simulink model "HQEV_MiL_20160830_integrate_2010a"  (Simulink 7.5)
settings: Solver=FixedStepDiscrete  StartTime=0.0  StopTime=inf  FixedStep=0.01  RelTol=1e-3
PostLoadFcn:
  | , if any(exist('dsrtsu_mdlpostloadfcn', 'file') == [2, 3, 6]), try dsrtsu_mdlpostloadfcn('Execute', bdroot); catch fprintf('Error in PostLoadFcn (dsrtsu_mdlpostloadfcn) for model "%s":\n %s\n', bdroot, lasterr); end, end,
values from neighbouring files (symbols this model uses):
  Bat_C_Ah = 36    [parameter_V1.mat]
  Bat_ocv_xIndex = [5 10 20 30 40 50 60 70 80 90 95]    [parameter_V1.mat]
  Bat_ocv_z = [329 332 340 345 347 351 358 372 377 386 391]    [parameter_V1.mat]
  Bat_R_ohm_z = [4.41 3.46 1.57 1.07 0.76 0.63 0.55 0.44 0.41 0.4 0.4 3.14 ... (66 elements, 11x6)]    [parameter_V1.mat]
  Bat_SOC_Init = 90    [parameter_V1.mat]
  Env_hum_pct_Ambient = 30    [parameter_V1.mat]
  Env_Slope_deg = 0    [parameter_V1.mat]
  Env_Temp_degC_Ambient = 25    [parameter_V1.mat]
  Env_v_kmph_HWind = 0    [parameter_V1.mat]
  Reducer_F_i = 7.23    [parameter_V1.mat]
  Reducer_R_i = 7.23    [parameter_V1.mat]
  Veh =     [parameter_V1.mat]
  Veh_A_m2_Fr = 2.246    [parameter_V1.mat]
  Veh_F_Brake =     [parameter_V1.mat]
  Veh_fac_AirDrag = 0.326    [parameter_V1.mat]
  Veh_fac_WhDragFrict_0 = 0.011    [parameter_V1.mat]
  Veh_g_mps2_C = 9.81    [parameter_V1.mat]
  Veh_GainBrake =     [parameter_V1.mat]
  Veh_h_m_COGHigh = 0.5    [parameter_V1.mat]
  Veh_J_kgm2_Wh = 1.3635    [parameter_V1.mat]
  Veh_L_m_AxlBas = 2.63    [parameter_V1.mat]
  Veh_M_kg = 1427    [parameter_V1.mat]
  Veh_mu_Brake = 0.4    [parameter_V1.mat]
  Veh_mu_Tyre =     [parameter_V1.mat]
  Veh_num_FrictPair = 8    [parameter_V1.mat]
  Veh_pct_Brk = 70    [parameter_V1.mat]
  Veh_r_dyn =     [parameter_V1.mat]
  Veh_r_m_BrkDisk = 0.136    [parameter_V1.mat]
  Veh_rho_kgpm3_Air = 1.2258    [parameter_V1.mat]
undefined symbols (not defined in the file or in its folder): DiscIntNeverNeededParam, p_bool_False_M, p_bool_True_M
libraries: BaseOperationLib_Browser x38, simulink x14, DTQC_lib x1, ERR_lib x1, MQM_lib x1, PTCL_lib x1, PUD_lib x1, TQD_lib x1, TQR_lib x1, VMM_lib x1, ACCA_lib x1, BBCA_lib x1
(part 14 of 15)

== system HQEV_MiL_20160830_integrate_2010a/MiL/Test_Integration/Reducer_R/FinalDrive/FinalDrive/Subsystem/Backward/Efficiency ==
  T_in : Inport
  "Temp " : Inport  Port=2
  "Omega_in " : Inport  Port=3
  Terminator : Terminator
  Terminator1 : Terminator
  Terminator2 : Terminator
  eta_constant : Constant  Value=0.94
  eta : Outport
  wires:
  "Temp "/1 -> Terminator2/1
  T_in/1 -> Terminator1/1
  "Omega_in "/1 -> Terminator/1
  eta_constant/1 -> eta/1

== system HQEV_MiL_20160830_integrate_2010a/MiL/Test_Integration/Reducer_R/FinalDrive/FinalDrive/Subsystem/Forward/Efficiency ==
  T_in : Inport
  "Temp " : Inport  Port=2
  "Omega_in " : Inport  Port=3
  Terminator : Terminator
  Terminator1 : Terminator
  Terminator2 : Terminator
  eta_constant : Constant  Value=0.94
  eta : Outport
  wires:
  "Temp "/1 -> Terminator2/1
  T_in/1 -> Terminator1/1
  "Omega_in "/1 -> Terminator/1
  eta_constant/1 -> eta/1

== system HQEV_MiL_20160830_integrate_2010a/MiL/Test_Integration/Thermal/Thermal/Subsystem/Battery_Cooling_Circle/Battery/Forced Convective ==
  note: C:specific heat capacity
  note: CQ(T2-T1)=h[T0-(T2+T1)/2]
      | T2=(hT0+CQT1-T1h/2)/(CQ+h/2)
  note: h: forced convective heat transfer coefficient
  T_Motor : Inport
  Q_water_inlet : Inport  Port=2
  T_water_inlet : Inport  Port=3
  Bus Creator : BusCreator  Inputs=5
  Bus Selector : BusSelector  OutputSignals=T_Motor,h
  Bus Selector1 : BusSelector  OutputSignals=T_Water_Inlet,Q_Water_Inlet,C
  Bus Selector2 : BusSelector  OutputSignals=T_Water_Inlet,h
  Bus Selector3 : BusSelector  OutputSignals=Q_Water_Inlet,C,h
  Bus Selector4 : BusSelector  OutputSignals=Q_Water_Inlet,C,T_Water_Inlet
  C : Constant  Value=3400
  CQT{1..8} (8 alike) : Product  RndMeth=Zero
  Const1 : Constant  Value=0.5
  Const2 : Constant  Value=0.5
  Divide1 : Product  Inputs=*/
  Scope1 : Scope
      settings: TimeRange=40  YMin=-1  YMax=1  SaveName=ScopeData22
  Scope5 : Scope
      settings: TimeRange=40  YMin=-1  YMax=1  SaveName=ScopeData21
  Subtract1 : Sum  Inputs=+-
  Subtract2 : Sum  Inputs=+-
  Unit Delay : UnitDelay  SampleTime=-1
  add2 : Sum
  add3 : Sum
  h W/deg : Constant  Value=500
  hT0 : Product  RndMeth=Zero
  q_Water2Motor : Outport
  T_water_outlet : Outport  Port=2
  Q_water_outlet : Outport  Port=3
  wires:
  T_Motor/1 -> Bus Creator/2  "T_Motor"
  T_water_inlet/1 -> Bus Creator/1  "T_Water_Inlet"
  Q_water_inlet/1 -> Bus Creator/3, Q_water_outlet/1  "Q_Water_Inlet"
  h W/deg/1 -> Bus Creator/4  "h"
  C/1 -> Bus Creator/5  "C"
  Bus Creator/1 -> Bus Selector/1, Bus Selector1/1, Bus Selector2/1, Bus Selector3/1, Bus Selector4/1
  Bus Selector/1 -> hT0/1  "<T_Motor>"
  Bus Selector/2 -> hT0/2  "<h>"
  Bus Selector1/1 -> CQT1/1  "<T_Water_Inlet>"
  Bus Selector1/2 -> CQT1/2  "<Q_Water_Inlet>"
  CQT1/1 -> CQT2/1
  Bus Selector1/3 -> CQT2/2  "<C>"
  Bus Selector2/1 -> CQT3/1  "<T_Water_Inlet>"
  Bus Selector2/2 -> CQT3/2  "<h>"
  CQT3/1 -> CQT4/1
  Const2/1 -> CQT4/2
  hT0/1 -> add2/1
  CQT2/1 -> add2/2
  add2/1 -> Subtract1/1
  CQT4/1 -> Subtract1/2
  Subtract1/1 -> Divide1/1
  Bus Selector3/1 -> CQT5/1  "<Q_Water_Inlet>"
  Bus Selector3/2 -> CQT5/2  "<C>"
  CQT5/1 -> add3/1
  Bus Selector3/3 -> CQT6/1  "<h>"
  Const1/1 -> CQT6/2
  CQT6/1 -> add3/2
  add3/1 -> Divide1/2
  Divide1/1 -> T_water_outlet/1, Unit Delay/1
  Bus Selector4/1 -> CQT7/1  "<Q_Water_Inlet>"
  Bus Selector4/2 -> CQT7/2  "<C>"
  Bus Selector4/3 -> Subtract2/1  "<T_Water_Inlet>"
  Unit Delay/1 -> Subtract2/2
  CQT7/1 -> CQT8/1, Scope5/1
  Subtract2/1 -> CQT8/2, Scope1/1
  CQT8/1 -> q_Water2Motor/1

== system HQEV_MiL_20160830_integrate_2010a/MiL/Test_Integration/Thermal/Thermal/Subsystem/Battery_Cooling_Circle/Battery/Free Convective ==
  Q_water_inlet : Inport
  T_water_inlet : Inport  Port=2
  T_water_outlet : Outport
  Q_water_outlet : Outport  Port=2
  wires:
  Q_water_inlet/1 -> Q_water_outlet/1
  T_water_inlet/1 -> T_water_outlet/1

== system HQEV_MiL_20160830_integrate_2010a/MiL/Test_Integration/Thermal/Thermal/Subsystem/Battery_Cooling_Circle/Battery/Thermal_Mass ==
  note: h: forced convective heat transfer coefficient
  note: CQ(T2-T1)=h[T0-(T2+T1)/2]
      | T2=(hT0+CQT1-T1h/2)/(CQ+h/2)
  note: C:specific heat capacity
  pwr_MotorLoss : Inport
  pwr_Water2Motor : Inport  Port=2
  BatTempIndex : Inport  Port=3
  Add : Sum
  Add1 : Sum
  C J/kg/deg : Constant  Value=450
  Compare To Constant : simulink/Logic and Bit Operations/Compare To Constant  SystemSampleTime=-1  relop===  const=0  LogicOutDataTypeMode=boolean
  Discrete-Time Integrator : DiscreteIntegrator  SampleTime=0.01  ICPrevOutput=DiscIntNeverNeededParam  ICPrevScaledInput=DiscIntNeverNeededParam
  Divide : Product  Inputs=*/
  Divide1 : Product  Inputs=*/
  Init_temp : Constant  Value=20
  Scope{,1..7} (8 alike) : Scope
      Scope settings: YMin=-1.05  YMax=-0.95  SaveName=ScopeData5
      Scope1 settings: YMin=-1.05  YMax=-0.95  SaveName=ScopeData13
      Scope2 settings: YMin=-1.05  YMax=-0.95  SaveName=ScopeData14
      Scope3 settings: YMin=-1.05  YMax=-0.95  SaveName=ScopeData15
      Scope4 settings: YMin=-1.05  YMax=-0.95  SaveName=ScopeData18
      Scope5 settings: YMin=-1.05  YMax=-0.95  SaveName=ScopeData19
      Scope6 settings: YMin=2.0625  YMax=2.11  SaveName=ScopeData20
      Scope7 settings: YMin=-1.05  YMax=-0.95  SaveName=ScopeData12
  Switch : Switch  Criteria=u2 > Threshold
  m kg : Constant  Value=200
  T_Motor : Outport
  wires:
  pwr_Water2Motor/1 -> Add/1, Scope4/1
  pwr_MotorLoss/1 -> Add/2, Scope5/1
  Add/1 -> Discrete-Time Integrator/1, Scope3/1
  Discrete-Time Integrator/1 -> Divide/1, Scope2/1
  C J/kg/deg/1 -> Divide/2
  Divide/1 -> Divide1/1, Scope1/1
  m kg/1 -> Divide1/2
  Divide1/1 -> Add1/1, Scope6/1
  Add1/1 -> T_Motor/1, Scope7/1
  BatTempIndex/1 -> Switch/3, Compare To Constant/1
  Compare To Constant/1 -> Switch/2
  Switch/1 -> Add1/2, Scope/1
  Init_temp/1 -> Switch/1

== system HQEV_MiL_20160830_integrate_2010a/MiL/Test_Integration/Thermal/Thermal/Subsystem/Battery_Cooling_Circle/Chiller/Forced Convective ==
  note: C:specific heat capacity
  note: CQ(T1-T2)=P
  note: h: forced convective heat transfer coefficient
  AC_OnOff : Inport
  Q_water_inlet : Inport  Port=2
  Temp_water_inlet : Inport  Port=3
  C J/kg/deg : Constant  Value=3400
  Divide : Product  Inputs=*/
  Product : Product  RndMeth=Zero
  Product1 : Product  RndMeth=Zero
  Saturation : Saturate  UpperLimit=inf  LowerLimit=0.5
  Subtract : Sum  Inputs=+-
  Unit Delay : UnitDelay  SampleTime=-1
  pwr_Chiller : Constant  Value=3000
  T_water_outlet : Outport
  Q_water_outlet : Outport  Port=2
  wires:
  Unit Delay/1 -> Q_water_outlet/1, Product/2
  Q_water_inlet/1 -> Unit Delay/1
  C J/kg/deg/1 -> Product/1
  Product/1 -> Saturation/1
  AC_OnOff/1 -> Product1/1
  pwr_Chiller/1 -> Product1/2
  Saturation/1 -> Divide/2
  Product1/1 -> Divide/1
  Divide/1 -> Subtract/2
  Temp_water_inlet/1 -> Subtract/1
  Subtract/1 -> T_water_outlet/1

== system HQEV_MiL_20160830_integrate_2010a/MiL/Test_Integration/Thermal/Thermal/Subsystem/Battery_Cooling_Circle/Chiller/Free Convective ==
  Q_water_inlet : Inport
  T_water_inlet : Inport  Port=2
  T_water_outlet : Outport
  Q_water_outlet : Outport  Port=2
  wires:
  Q_water_inlet/1 -> Q_water_outlet/1
  T_water_inlet/1 -> T_water_outlet/1

== system HQEV_MiL_20160830_integrate_2010a/MiL/Test_Integration/Thermal/Thermal/Subsystem/Battery_Cooling_Circle/PTC/Forced Convective ==
  note: C:specific heat capacity
  note: CQ(T1-T2)=P
  note: h: forced convective heat transfer coefficient
  PWM_PTC_pct : Inport
  Q_water_inlet : Inport  Port=2
  Temp_water_inlet : Inport  Port=3
  C : Constant
  Divide : Product  Inputs=*/
  Product : Product  RndMeth=Zero
  Product1 : Product  RndMeth=Zero
  Product2 : Product  RndMeth=Zero
  Saturation : Saturate  UpperLimit=inf  LowerLimit=0.5
  Subtract : Sum  Inputs=+-
  Unit Delay : UnitDelay  SampleTime=-1
  pct : Constant  Value=0.01
  pwr_PTC : Constant  Value=3000
  T_water_outlet : Outport
  Q_water_outlet : Outport  Port=2
  wires:
  Unit Delay/1 -> Q_water_outlet/1, Product/2
  Q_water_inlet/1 -> Unit Delay/1
  C/1 -> Product/1
  Product/1 -> Saturation/1
  pwr_PTC/1 -> Product1/2
  Saturation/1 -> Divide/2
  Product1/1 -> Divide/1
  Divide/1 -> Subtract/2
  Temp_water_inlet/1 -> Subtract/1
  Subtract/1 -> T_water_outlet/1
  PWM_PTC_pct/1 -> Product2/1
  pct/1 -> Product2/2
  Product2/1 -> Product1/1

== system HQEV_MiL_20160830_integrate_2010a/MiL/Test_Integration/Thermal/Thermal/Subsystem/Battery_Cooling_Circle/PTC/Free Convective ==
  Q_water_inlet : Inport
  T_water_inlet : Inport  Port=2
  T_water_outlet : Outport
  Q_water_outlet : Outport  Port=2
  wires:
  Q_water_inlet/1 -> Q_water_outlet/1
  T_water_inlet/1 -> T_water_outlet/1

== system HQEV_MiL_20160830_integrate_2010a/MiL/Test_Integration/Thermal/Thermal/Subsystem/Motor_Cooling_Circle/Charger/Forced Convective ==
  note: C:specific heat capacity
  note: CQ(T2-T1)=h[T0-(T2+T1)/2]
      | T2=(hT0+CQT1-T1h/2)/(CQ+h/2)
  note: h: forced convective heat transfer coefficient
  T_Motor : Inport
  Q_water_inlet : Inport  Port=2
  T_water_inlet : Inport  Port=3
  Bus Creator : BusCreator  Inputs=5
  Bus Selector : BusSelector  OutputSignals=T_Motor,h
  Bus Selector1 : BusSelector  OutputSignals=T_Water_Inlet,Q_Water_Inlet,C
  Bus Selector2 : BusSelector  OutputSignals=T_Water_Inlet,h
  Bus Selector3 : BusSelector  OutputSignals=Q_Water_Inlet,C,h
  Bus Selector4 : BusSelector  OutputSignals=Q_Water_Inlet,C,T_Water_Inlet
  C : Constant  Value=3400
  CQT{1..8} (8 alike) : Product  RndMeth=Zero
  Const1 : Constant  Value=0.5
  Const2 : Constant  Value=0.5
  Divide1 : Product  Inputs=*/
  Subtract1 : Sum  Inputs=+-
  Subtract2 : Sum  Inputs=+-
  Unit Delay : UnitDelay  SampleTime=-1
  add2 : Sum
  add3 : Sum
  h W/deg : Constant  Value=500
  hT0 : Product  RndMeth=Zero
  q_Water2Motor : Outport
  T_water_outlet : Outport  Port=2
  Q_water_outlet : Outport  Port=3
  wires:
  T_Motor/1 -> Bus Creator/2  "T_Motor"
  T_water_inlet/1 -> Bus Creator/1  "T_Water_Inlet"
  Q_water_inlet/1 -> Bus Creator/3, Q_water_outlet/1  "Q_Water_Inlet"
  h W/deg/1 -> Bus Creator/4  "h"
  C/1 -> Bus Creator/5  "C"
  Bus Creator/1 -> Bus Selector/1, Bus Selector1/1, Bus Selector2/1, Bus Selector3/1, Bus Selector4/1
  Bus Selector/1 -> hT0/1  "<T_Motor>"
  Bus Selector/2 -> hT0/2  "<h>"
  Bus Selector1/1 -> CQT1/1  "<T_Water_Inlet>"
  Bus Selector1/2 -> CQT1/2  "<Q_Water_Inlet>"
  CQT1/1 -> CQT2/1
  Bus Selector1/3 -> CQT2/2  "<C>"
  Bus Selector2/1 -> CQT3/1  "<T_Water_Inlet>"
  Bus Selector2/2 -> CQT3/2  "<h>"
  CQT3/1 -> CQT4/1
  Const2/1 -> CQT4/2
  hT0/1 -> add2/1
  CQT2/1 -> add2/2
  add2/1 -> Subtract1/1
  CQT4/1 -> Subtract1/2
  Subtract1/1 -> Divide1/1
  Bus Selector3/1 -> CQT5/1  "<Q_Water_Inlet>"
  Bus Selector3/2 -> CQT5/2  "<C>"
  CQT5/1 -> add3/1
  Bus Selector3/3 -> CQT6/1  "<h>"
  Const1/1 -> CQT6/2
  CQT6/1 -> add3/2
  add3/1 -> Divide1/2
  Divide1/1 -> T_water_outlet/1, Unit Delay/1
  Bus Selector4/1 -> CQT7/1  "<Q_Water_Inlet>"
  Bus Selector4/2 -> CQT7/2  "<C>"
  Bus Selector4/3 -> Subtract2/1  "<T_Water_Inlet>"
  Unit Delay/1 -> Subtract2/2
  CQT7/1 -> CQT8/1
  Subtract2/1 -> CQT8/2
  CQT8/1 -> q_Water2Motor/1

== system HQEV_MiL_20160830_integrate_2010a/MiL/Test_Integration/Thermal/Thermal/Subsystem/Motor_Cooling_Circle/Charger/Free Convective ==
  Q_water_inlet : Inport
  T_water_inlet : Inport  Port=2
  T_water_outlet : Outport
  Q_water_outlet : Outport  Port=2
  wires:
  Q_water_inlet/1 -> Q_water_outlet/1
  T_water_inlet/1 -> T_water_outlet/1

== system HQEV_MiL_20160830_integrate_2010a/MiL/Test_Integration/Thermal/Thermal/Subsystem/Motor_Cooling_Circle/Charger/Thermal_Mass ==
  note: h: forced convective heat transfer coefficient
  note: CQ(T2-T1)=h[T0-(T2+T1)/2]
      | T2=(hT0+CQT1-T1h/2)/(CQ+h/2)
  note: C:specific heat capacity
  pwr_MotorLoss : Inport
  pwr_Water2Motor : Inport  Port=2
  Add : Sum
  Add1 : Sum
  C J/kg/deg : Constant  Value=450
  Discrete-Time Integrator : DiscreteIntegrator  SampleTime=0.01  ICPrevOutput=DiscIntNeverNeededParam  ICPrevScaledInput=DiscIntNeverNeededParam
  Divide : Product  Inputs=*/
  Divide1 : Product  Inputs=*/
  Init_temp : Constant  Value=20
  m kg : Constant  Value=5
  T_Motor : Outport
  wires:
  pwr_Water2Motor/1 -> Add/1
  pwr_MotorLoss/1 -> Add/2
  Add/1 -> Discrete-Time Integrator/1
  Discrete-Time Integrator/1 -> Divide/1
  C J/kg/deg/1 -> Divide/2
  Divide/1 -> Divide1/1
  m kg/1 -> Divide1/2
  Divide1/1 -> Add1/1
  Init_temp/1 -> Add1/2
  Add1/1 -> T_Motor/1

== system HQEV_MiL_20160830_integrate_2010a/MiL/Test_Integration/Thermal/Thermal/Subsystem/Motor_Cooling_Circle/DCDC/Forced Convective ==
  note: C:specific heat capacity
  note: CQ(T2-T1)=h[T0-(T2+T1)/2]
      | T2=(hT0+CQT1-T1h/2)/(CQ+h/2)
  note: h: forced convective heat transfer coefficient
  T_Motor : Inport
  Q_water_inlet : Inport  Port=2
  T_water_inlet : Inport  Port=3
  Bus Creator : BusCreator  Inputs=5
  Bus Selector : BusSelector  OutputSignals=T_Motor,h
  Bus Selector1 : BusSelector  OutputSignals=T_Water_Inlet,Q_Water_Inlet,C
  Bus Selector2 : BusSelector  OutputSignals=T_Water_Inlet,h
  Bus Selector3 : BusSelector  OutputSignals=Q_Water_Inlet,C,h
  Bus Selector4 : BusSelector  OutputSignals=Q_Water_Inlet,C,T_Water_Inlet
  C : Constant  Value=3400
  CQT{1..8} (8 alike) : Product  RndMeth=Zero
  Const1 : Constant  Value=0.5
  Const2 : Constant  Value=0.5
  Divide1 : Product  Inputs=*/
  Subtract1 : Sum  Inputs=+-
  Subtract2 : Sum  Inputs=+-
  Unit Delay : UnitDelay  SampleTime=-1
  add2 : Sum
  add3 : Sum
  h W/deg : Constant  Value=500
  hT0 : Product  RndMeth=Zero
  q_Water2Motor : Outport
  T_water_outlet : Outport  Port=2
  Q_water_outlet : Outport  Port=3
  wires:
  T_Motor/1 -> Bus Creator/2  "T_Motor"
  T_water_inlet/1 -> Bus Creator/1  "T_Water_Inlet"
  Q_water_inlet/1 -> Bus Creator/3, Q_water_outlet/1  "Q_Water_Inlet"
  h W/deg/1 -> Bus Creator/4  "h"
  C/1 -> Bus Creator/5  "C"
  Bus Creator/1 -> Bus Selector/1, Bus Selector1/1, Bus Selector2/1, Bus Selector3/1, Bus Selector4/1
  Bus Selector/1 -> hT0/1  "<T_Motor>"
  Bus Selector/2 -> hT0/2  "<h>"
  Bus Selector1/1 -> CQT1/1  "<T_Water_Inlet>"
  Bus Selector1/2 -> CQT1/2  "<Q_Water_Inlet>"
  CQT1/1 -> CQT2/1
  Bus Selector1/3 -> CQT2/2  "<C>"
  Bus Selector2/1 -> CQT3/1  "<T_Water_Inlet>"
  Bus Selector2/2 -> CQT3/2  "<h>"
  CQT3/1 -> CQT4/1
  Const2/1 -> CQT4/2
  hT0/1 -> add2/1
  CQT2/1 -> add2/2
  add2/1 -> Subtract1/1
  CQT4/1 -> Subtract1/2
  Subtract1/1 -> Divide1/1
  Bus Selector3/1 -> CQT5/1  "<Q_Water_Inlet>"
  Bus Selector3/2 -> CQT5/2  "<C>"
  CQT5/1 -> add3/1
  Bus Selector3/3 -> CQT6/1  "<h>"
  Const1/1 -> CQT6/2
  CQT6/1 -> add3/2
  add3/1 -> Divide1/2
  Divide1/1 -> T_water_outlet/1, Unit Delay/1
  Bus Selector4/1 -> CQT7/1  "<Q_Water_Inlet>"
  Bus Selector4/2 -> CQT7/2  "<C>"
  Bus Selector4/3 -> Subtract2/1  "<T_Water_Inlet>"
  Unit Delay/1 -> Subtract2/2
  CQT7/1 -> CQT8/1
  Subtract2/1 -> CQT8/2
  CQT8/1 -> q_Water2Motor/1

== system HQEV_MiL_20160830_integrate_2010a/MiL/Test_Integration/Thermal/Thermal/Subsystem/Motor_Cooling_Circle/DCDC/Free Convective ==
  Q_water_inlet : Inport
  T_water_inlet : Inport  Port=2
  T_water_outlet : Outport
  Q_water_outlet : Outport  Port=2
  wires:
  Q_water_inlet/1 -> Q_water_outlet/1
  T_water_inlet/1 -> T_water_outlet/1

== system HQEV_MiL_20160830_integrate_2010a/MiL/Test_Integration/Thermal/Thermal/Subsystem/Motor_Cooling_Circle/DCDC/Thermal_Mass ==
  note: h: forced convective heat transfer coefficient
  note: CQ(T2-T1)=h[T0-(T2+T1)/2]
      | T2=(hT0+CQT1-T1h/2)/(CQ+h/2)
  note: C:specific heat capacity
  pwr_MotorLoss : Inport
  pwr_Water2Motor : Inport  Port=2
  Add : Sum
  Add1 : Sum
  C J/kg/deg : Constant  Value=450
  Discrete-Time Integrator : DiscreteIntegrator  SampleTime=0.01  ICPrevOutput=DiscIntNeverNeededParam  ICPrevScaledInput=DiscIntNeverNeededParam
  Divide : Product  Inputs=*/
  Divide1 : Product  Inputs=*/
  Init_temp : Constant  Value=20
  m kg : Constant  Value=5
  T_Motor : Outport
  wires:
  pwr_Water2Motor/1 -> Add/1
  pwr_MotorLoss/1 -> Add/2
  Add/1 -> Discrete-Time Integrator/1
  Discrete-Time Integrator/1 -> Divide/1
  C J/kg/deg/1 -> Divide/2
  Divide/1 -> Divide1/1
  m kg/1 -> Divide1/2
  Divide1/1 -> Add1/1
  Init_temp/1 -> Add1/2
  Add1/1 -> T_Motor/1

== system HQEV_MiL_20160830_integrate_2010a/MiL/Test_Integration/Thermal/Thermal/Subsystem/Motor_Cooling_Circle/Motor_F/Forced Convective ==
  note: C:specific heat capacity
  note: CQ(T2-T1)=h[T0-(T2+T1)/2]
      | T2=(hT0+CQT1-T1h/2)/(CQ+h/2)
  note: h: forced convective heat transfer coefficient
  T_Motor : Inport
  Q_water_inlet : Inport  Port=2
  T_water_inlet : Inport  Port=3
  Bus Creator : BusCreator  Inputs=5
  Bus Selector : BusSelector  OutputSignals=T_Motor,h
  Bus Selector1 : BusSelector  OutputSignals=T_Water_Inlet,Q_Water_Inlet,C
  Bus Selector2 : BusSelector  OutputSignals=T_Water_Inlet,h
  Bus Selector3 : BusSelector  OutputSignals=Q_Water_Inlet,C,h
  Bus Selector4 : BusSelector  OutputSignals=Q_Water_Inlet,C,T_Water_Inlet
  C : Constant  Value=3400
  CQT{1..8} (8 alike) : Product  RndMeth=Zero
  Const1 : Constant  Value=0.5
  Const2 : Constant  Value=0.5
  Divide1 : Product  Inputs=*/
  Subtract1 : Sum  Inputs=+-
  Subtract2 : Sum  Inputs=+-
  Unit Delay : UnitDelay  SampleTime=-1
  add2 : Sum
  add3 : Sum
  h W/deg : Constant  Value=500
  hT0 : Product  RndMeth=Zero
  q_Water2Motor : Outport
  T_water_outlet : Outport  Port=2
  Q_water_outlet : Outport  Port=3
  wires:
  T_Motor/1 -> Bus Creator/2  "T_Motor"
  T_water_inlet/1 -> Bus Creator/1  "T_Water_Inlet"
  Q_water_inlet/1 -> Bus Creator/3, Q_water_outlet/1  "Q_Water_Inlet"
  h W/deg/1 -> Bus Creator/4  "h"
  C/1 -> Bus Creator/5  "C"
  Bus Creator/1 -> Bus Selector/1, Bus Selector1/1, Bus Selector2/1, Bus Selector3/1, Bus Selector4/1
  Bus Selector/1 -> hT0/1  "<T_Motor>"
  Bus Selector/2 -> hT0/2  "<h>"
  Bus Selector1/1 -> CQT1/1  "<T_Water_Inlet>"
  Bus Selector1/2 -> CQT1/2  "<Q_Water_Inlet>"
  CQT1/1 -> CQT2/1
  Bus Selector1/3 -> CQT2/2  "<C>"
  Bus Selector2/1 -> CQT3/1  "<T_Water_Inlet>"
  Bus Selector2/2 -> CQT3/2  "<h>"
  CQT3/1 -> CQT4/1
  Const2/1 -> CQT4/2
  hT0/1 -> add2/1
  CQT2/1 -> add2/2
  add2/1 -> Subtract1/1
  CQT4/1 -> Subtract1/2
  Subtract1/1 -> Divide1/1
  Bus Selector3/1 -> CQT5/1  "<Q_Water_Inlet>"
  Bus Selector3/2 -> CQT5/2  "<C>"
  CQT5/1 -> add3/1
  Bus Selector3/3 -> CQT6/1  "<h>"
  Const1/1 -> CQT6/2
  CQT6/1 -> add3/2
  add3/1 -> Divide1/2
  Divide1/1 -> T_water_outlet/1, Unit Delay/1
  Bus Selector4/1 -> CQT7/1  "<Q_Water_Inlet>"
  Bus Selector4/2 -> CQT7/2  "<C>"
  Bus Selector4/3 -> Subtract2/1  "<T_Water_Inlet>"
  Unit Delay/1 -> Subtract2/2
  CQT7/1 -> CQT8/1
  Subtract2/1 -> CQT8/2
  CQT8/1 -> q_Water2Motor/1

== system HQEV_MiL_20160830_integrate_2010a/MiL/Test_Integration/Thermal/Thermal/Subsystem/Motor_Cooling_Circle/Motor_F/Free Convective ==
  Q_water_inlet : Inport
  T_water_inlet : Inport  Port=2
  T_water_outlet : Outport
  Q_water_outlet : Outport  Port=2
  wires:
  Q_water_inlet/1 -> Q_water_outlet/1
  T_water_inlet/1 -> T_water_outlet/1

== system HQEV_MiL_20160830_integrate_2010a/MiL/Test_Integration/Thermal/Thermal/Subsystem/Motor_Cooling_Circle/Motor_F/Thermal_Mass ==
  note: h: forced convective heat transfer coefficient
  note: CQ(T2-T1)=h[T0-(T2+T1)/2]
      | T2=(hT0+CQT1-T1h/2)/(CQ+h/2)
  note: C:specific heat capacity
  pwr_MotorLoss : Inport
  pwr_Water2Motor : Inport  Port=2
  Add : Sum
  Add1 : Sum
  C J/kg/deg : Constant  Value=450
  Discrete-Time Integrator : DiscreteIntegrator  SampleTime=0.01  ICPrevOutput=DiscIntNeverNeededParam  ICPrevScaledInput=DiscIntNeverNeededParam
  Divide : Product  Inputs=*/
  Divide1 : Product  Inputs=*/
  Init_temp : Constant  Value=20
  m kg : Constant  Value=30
  T_Motor : Outport
  wires:
  pwr_Water2Motor/1 -> Add/1
  pwr_MotorLoss/1 -> Add/2
  Add/1 -> Discrete-Time Integrator/1
  Discrete-Time Integrator/1 -> Divide/1
  C J/kg/deg/1 -> Divide/2
  Divide/1 -> Divide1/1
  m kg/1 -> Divide1/2
  Divide1/1 -> Add1/1
  Init_temp/1 -> Add1/2
  Add1/1 -> T_Motor/1

== system HQEV_MiL_20160830_integrate_2010a/MiL/Test_Integration/Thermal/Thermal/Subsystem/Motor_Cooling_Circle/Motor_R/Forced Convective ==
  note: C:specific heat capacity
  note: CQ(T2-T1)=h[T0-(T2+T1)/2]
      | T2=(hT0+CQT1-T1h/2)/(CQ+h/2)
  note: h: forced convective heat transfer coefficient
  T_Motor : Inport
  Q_water_inlet : Inport  Port=2
  T_water_inlet : Inport  Port=3
  Bus Creator : BusCreator  Inputs=5
  Bus Selector : BusSelector  OutputSignals=T_Motor,h
  Bus Selector1 : BusSelector  OutputSignals=T_Water_Inlet,Q_Water_Inlet,C
  Bus Selector2 : BusSelector  OutputSignals=T_Water_Inlet,h
  Bus Selector3 : BusSelector  OutputSignals=Q_Water_Inlet,C,h
  Bus Selector4 : BusSelector  OutputSignals=Q_Water_Inlet,C,T_Water_Inlet
  C : Constant  Value=3400
  CQT{1..8} (8 alike) : Product  RndMeth=Zero
  Const1 : Constant  Value=0.5
  Const2 : Constant  Value=0.5
  Divide1 : Product  Inputs=*/
  Subtract1 : Sum  Inputs=+-
  Subtract2 : Sum  Inputs=+-
  Unit Delay : UnitDelay  SampleTime=-1
  add2 : Sum
  add3 : Sum
  h W/deg : Constant  Value=500
  hT0 : Product  RndMeth=Zero
  q_Water2Motor : Outport
  T_water_outlet : Outport  Port=2
  Q_water_outlet : Outport  Port=3
  wires:
  T_Motor/1 -> Bus Creator/2  "T_Motor"
  T_water_inlet/1 -> Bus Creator/1  "T_Water_Inlet"
  Q_water_inlet/1 -> Bus Creator/3, Q_water_outlet/1  "Q_Water_Inlet"
  h W/deg/1 -> Bus Creator/4  "h"
  C/1 -> Bus Creator/5  "C"
  Bus Creator/1 -> Bus Selector/1, Bus Selector1/1, Bus Selector2/1, Bus Selector3/1, Bus Selector4/1
  Bus Selector/1 -> hT0/1  "<T_Motor>"
  Bus Selector/2 -> hT0/2  "<h>"
  Bus Selector1/1 -> CQT1/1  "<T_Water_Inlet>"
  Bus Selector1/2 -> CQT1/2  "<Q_Water_Inlet>"
  CQT1/1 -> CQT2/1
  Bus Selector1/3 -> CQT2/2  "<C>"
  Bus Selector2/1 -> CQT3/1  "<T_Water_Inlet>"
  Bus Selector2/2 -> CQT3/2  "<h>"
  CQT3/1 -> CQT4/1
  Const2/1 -> CQT4/2
  hT0/1 -> add2/1
  CQT2/1 -> add2/2
  add2/1 -> Subtract1/1
  CQT4/1 -> Subtract1/2
  Subtract1/1 -> Divide1/1
  Bus Selector3/1 -> CQT5/1  "<Q_Water_Inlet>"
  Bus Selector3/2 -> CQT5/2  "<C>"
  CQT5/1 -> add3/1
  Bus Selector3/3 -> CQT6/1  "<h>"
  Const1/1 -> CQT6/2
  CQT6/1 -> add3/2
  add3/1 -> Divide1/2
  Divide1/1 -> T_water_outlet/1, Unit Delay/1
  Bus Selector4/1 -> CQT7/1  "<Q_Water_Inlet>"
  Bus Selector4/2 -> CQT7/2  "<C>"
  Bus Selector4/3 -> Subtract2/1  "<T_Water_Inlet>"
  Unit Delay/1 -> Subtract2/2
  CQT7/1 -> CQT8/1
  Subtract2/1 -> CQT8/2
  CQT8/1 -> q_Water2Motor/1

== system HQEV_MiL_20160830_integrate_2010a/MiL/Test_Integration/Thermal/Thermal/Subsystem/Motor_Cooling_Circle/Motor_R/Free Convective ==
  Q_water_inlet : Inport
  T_water_inlet : Inport  Port=2
  T_water_outlet : Outport
  Q_water_outlet : Outport  Port=2
  wires:
  Q_water_inlet/1 -> Q_water_outlet/1
  T_water_inlet/1 -> T_water_outlet/1

== system HQEV_MiL_20160830_integrate_2010a/MiL/Test_Integration/Thermal/Thermal/Subsystem/Motor_Cooling_Circle/Motor_R/Thermal_Mass ==
  note: h: forced convective heat transfer coefficient
  note: CQ(T2-T1)=h[T0-(T2+T1)/2]
      | T2=(hT0+CQT1-T1h/2)/(CQ+h/2)
  note: C:specific heat capacity
  pwr_MotorLoss : Inport
  pwr_Water2Motor : Inport  Port=2
  Add : Sum
  Add1 : Sum
  C J/kg/deg : Constant  Value=450
  Discrete-Time Integrator : DiscreteIntegrator  SampleTime=0.01  ICPrevOutput=DiscIntNeverNeededParam  ICPrevScaledInput=DiscIntNeverNeededParam
  Divide : Product  Inputs=*/
  Divide1 : Product  Inputs=*/
  Init_temp : Constant  Value=20
  m kg : Constant  Value=30
  T_Motor : Outport
  wires:
  pwr_Water2Motor/1 -> Add/1
  pwr_MotorLoss/1 -> Add/2
  Add/1 -> Discrete-Time Integrator/1
  Discrete-Time Integrator/1 -> Divide/1
  C J/kg/deg/1 -> Divide/2
  Divide/1 -> Divide1/1
  m kg/1 -> Divide1/2
  Divide1/1 -> Add1/1
  Init_temp/1 -> Add1/2
  Add1/1 -> T_Motor/1

== system HQEV_MiL_20160830_integrate_2010a/MiL/Test_Integration/Thermal/Thermal/Subsystem/Motor_Cooling_Circle/Radiator/Forced Convective ==
  note: h: forced convective heat transfer coefficient
  note: CQ(T2-T1)=h[T0-(T2+T1)/2]
      | T2=(hT0+CQT1-T1h/2)/(CQ+h/2)
  note: C:specific heat capacity
  PWM_Fan : Inport
  Q_water_inlet : Inport  Port=2
  T_water_inlet : Inport  Port=3
  Bus Creator : BusCreator  Inputs=5
  Bus Selector : BusSelector  OutputSignals=T_Motor,h
  Bus Selector1 : BusSelector  OutputSignals=T_Water_Inlet,Q_Water_Inlet,C
  Bus Selector2 : BusSelector  OutputSignals=T_Water_Inlet,h
  Bus Selector3 : BusSelector  OutputSignals=Q_Water_Inlet,C,h
  C J/kg/deg : Constant  Value=3400
  CQT{1..8} (8 alike) : Product  RndMeth=Zero
  Const1 : Constant  Value=0.5
  Const2 : Constant  Value=0.5
  Const3 : Constant  Value=0.01
  Divide1 : Product  Inputs=*/
  Env_Temp_Air : Constant  Value=25
  Saturation : Saturate  UpperLimit=inf  LowerLimit=0.1
  Subtract1 : Sum  Inputs=+-
  add2 : Sum
  add3 : Sum
  h W/deg : Constant  Value=3000
  hT0 : Product  RndMeth=Zero
  T_water_outlet : Outport
  Q_water_outlet : Outport  Port=2
  wires:
  Divide1/1 -> T_water_outlet/1
  add3/1 -> Saturation/1
  CQT6/1 -> add3/2
  Const1/1 -> CQT6/2
  Bus Selector3/3 -> CQT6/1  "<h>"
  CQT5/1 -> add3/1
  Bus Selector3/2 -> CQT5/2  "<C>"
  Bus Selector3/1 -> CQT5/1  "<Q_Water_Inlet>"
  Subtract1/1 -> Divide1/1
  CQT4/1 -> Subtract1/2
  add2/1 -> Subtract1/1
  CQT2/1 -> add2/2
  hT0/1 -> add2/1
  Const2/1 -> CQT4/2
  CQT3/1 -> CQT4/1
  Bus Selector2/2 -> CQT3/2  "<h>"
  Bus Selector2/1 -> CQT3/1  "<T_Water_Inlet>"
  Bus Selector1/3 -> CQT2/2  "<C>"
  CQT1/1 -> CQT2/1
  Bus Selector1/2 -> CQT1/2  "<Q_Water_Inlet>"
  Bus Selector1/1 -> CQT1/1  "<T_Water_Inlet>"
  Bus Selector/2 -> hT0/2  "<h>"
  Bus Selector/1 -> hT0/1  "<T_Motor>"
  Bus Creator/1 -> Bus Selector2/1, Bus Selector3/1, Bus Selector1/1, Bus Selector/1
  C J/kg/deg/1 -> Bus Creator/5  "C"
  Q_water_inlet/1 -> Bus Creator/3, Q_water_outlet/1  "Q_Water_Inlet"
  T_water_inlet/1 -> Bus Creator/1  "T_Water_Inlet"
  Env_Temp_Air/1 -> Bus Creator/2  "T_Motor"
  PWM_Fan/1 -> CQT7/1
  Const3/1 -> CQT7/2
  CQT7/1 -> CQT8/1
  h W/deg/1 -> CQT8/2
  CQT8/1 -> Bus Creator/4  "h"
  Saturation/1 -> Divide1/2

== system HQEV_MiL_20160830_integrate_2010a/MiL/Test_Integration/Thermal/Thermal/Subsystem/Motor_Cooling_Circle/Radiator/Free Convective ==
  Q_water_inlet : Inport
  T_water_inlet : Inport  Port=2
  T_water_outlet : Outport
  Q_water_outlet : Outport  Port=2
  wires:
  Q_water_inlet/1 -> Q_water_outlet/1
  T_water_inlet/1 -> T_water_outlet/1

== system HQEV_MiL_20160830_integrate_2010a/MiL/Test_Integration/Vehicle/Vehicle/Vehicle/Wheel Torque/maximal_wheel_torque/F_to_T ==
  F_normal [N] : Inport
  mu_Tyre : Gain  Gain=Veh_mu_Tyre.z  SaturateOnIntegerOverflow=on  OutDataTypeStr=Inherit: Same as input  ParamDataTypeStr=Inherit: Same as input
  r_dyn : Gain  Gain=Veh_r_dyn.z  SaturateOnIntegerOverflow=on  OutDataTypeStr=Inherit: Same as input  ParamDataTypeStr=Inherit: Same as input
  T_max [Nm] : Outport
  wires:
  mu_Tyre/1 -> r_dyn/1
  F_normal [N]/1 -> mu_Tyre/1
  r_dyn/1 -> T_max [Nm]/1

== system HQEV_MiL_20160830_integrate_2010a/MiL/Test_Integration/Vehicle/Vehicle/Vehicle/Wheel Torque/maximal_wheel_torque/F_to_T_ ==
  F_normal [N] : Inport
  mu_Tyre : Gain  Gain=Veh_mu_Tyre.z  SaturateOnIntegerOverflow=on  OutDataTypeStr=Inherit: Same as input  ParamDataTypeStr=Inherit: Same as input
  r_dyn : Gain  Gain=Veh_r_dyn.z  SaturateOnIntegerOverflow=on  OutDataTypeStr=Inherit: Same as input  ParamDataTypeStr=Inherit: Same as input
  T_max [Nm] : Outport
  wires:
  r_dyn/1 -> T_max [Nm]/1
  F_normal [N]/1 -> mu_Tyre/1
  mu_Tyre/1 -> r_dyn/1

== system HQEV_MiL_20160830_integrate_2010a/MiL/Test_Integration/Vehicle/Vehicle/Vehicle/Wheel Torque/maximal_wheel_torque/Normal_force ==
  note: COG to front axle
  note: COG to rear axle
  note: COG to ground
  note: gravity aceleration
  note: wheel base
  acc_Vehicle [m/s^2] : Inport
  phi_Slope [deg] : Inport  Port=2
  m [kg] : Inport  Port=3
  Add : Sum  Inputs=+-
  Add1 : Sum
  Add2 : Sum
  Constant1 : Constant  Value=Veh_g_mps2_C
  Constant4 : Constant  Value=Veh_L_m_AxlBas
  Constant5 : Constant  Value=Veh.L_m_COGFr
  Constant6 : Constant  Value=Veh.L_m_COGRear
  Constant7 : Constant  Value=Veh_h_m_COGHigh
  Divide1 : Product  Inputs=/***
  Divide2 : Product  Inputs=/**
  Divide3 : Product  Inputs=/***
  Product : Product  RndMeth=Zero
  Product1 : Product  RndMeth=Zero
  Product2 : Product  RndMeth=Zero
  Trigonometric Function : Trigonometry  Operator=cos
  Trigonometric Function1 : Trigonometry
  deg_rad : Gain  Gain=pi/180  SaturateOnIntegerOverflow=on  OutDataTypeStr=Inherit: Same as input  ParamDataTypeStr=Inherit: Same as input
  F_normalFront [N] : Outport
  F_normalRear [N] : Outport  Port=2
  wires:
  Product2/1 -> Add2/1
  Trigonometric Function1/1 -> Product2/2
  Add2/1 -> Divide2/3
  Constant4/1 -> Divide1/1, Divide2/1, Divide3/1
  Constant6/1 -> Divide3/2
  Constant5/1 -> Divide1/2
  Constant7/1 -> Divide2/2
  acc_Vehicle [m/s^2]/1 -> Add2/2
  Constant1/1 -> Product2/1, Divide1/3, Divide3/3
  Divide1/1 -> Add1/1
  Divide2/1 -> Add/2, Add1/2
  Divide3/1 -> Add/1
  Add1/1 -> Product/2
  Add/1 -> Product1/2
  Product/1 -> F_normalRear [N]/1
  Product1/1 -> F_normalFront [N]/1
  Trigonometric Function/1 -> Divide1/4, Divide3/4
  deg_rad/1 -> Trigonometric Function1/1, Trigonometric Function/1
  phi_Slope [deg]/1 -> deg_rad/1
  m [kg]/1 -> Product/1, Product1/1

== system HQEV_MiL_20160830_integrate_2010a/MiL/Test_Integration/Charger/Charger/Charger/Charger/Work/Subsystem/AC_Charge ==
  HCU_ChargePermission : Inport
  BMS_MainPosContactorState : Inport  Port=2
  HCU_ChargeHeatingPermission : Inport  Port=3
  BMS_MainNegContactorState : Inport  Port=4
  BMS_PreChargeContactorState : Inport  Port=5
  BMS_ChargePosContactorState : Inport  Port=6
  BMS_ChargeNegContactorState : Inport  Port=7
  Bus Creator : BusCreator  Inputs=2
  Bus Creator1 : BusCreator  Inputs=2
  Bus Creator2 : BusCreator  Inputs=2
  Bus Selector : BusSelector  OutputSignals=signal1,signal2
  Charger_I : Constant  Value=0
  Charger_I1 : Constant  Value=10
  Charger_I2 : Constant  Value=5
  Charger_U : Constant  Value=0
  Charger_U1 : Constant  Value=360
  Charger_U2 : Constant  Value=360
  Logical Operator : Logic  Operator=OR  AllPortsSameDT=off  OutDataTypeMode=boolean  OutDataTypeStr=boolean
  Logical Operator1 : Logic  AllPortsSameDT=off  OutDataTypeMode=boolean  OutDataTypeStr=boolean
  Logical Operator3 : Logic  AllPortsSameDT=off  OutDataTypeMode=boolean  OutDataTypeStr=boolean
  Switch : Switch  Criteria=u2 ~= 0
  Switch1 : Switch  Criteria=u2 ~= 0
  Terminator : Terminator
  Terminator1 : Terminator
  Terminator2 : Terminator
  ChargerOutputVoltage : Outport
  ChargerOutputCurrent : Outport  Port=2
  wires:
  BMS_PreChargeContactorState/1 -> Terminator/1
  BMS_ChargePosContactorState/1 -> Terminator1/1
  BMS_ChargeNegContactorState/1 -> Terminator2/1
  HCU_ChargePermission/1 -> Logical Operator/1, Logical Operator3/2
  HCU_ChargeHeatingPermission/1 -> Logical Operator/2
  Logical Operator/1 -> Switch/2
  Charger_U/1 -> Bus Creator/1
  Charger_I/1 -> Bus Creator/2
  Bus Creator/1 -> Switch/3
  BMS_MainPosContactorState/1 -> Logical Operator1/1
  BMS_MainNegContactorState/1 -> Logical Operator1/2
  Logical Operator1/1 -> Logical Operator3/1
  Logical Operator3/1 -> Switch1/2
  Charger_U1/1 -> Bus Creator1/1
  Charger_I1/1 -> Bus Creator1/2
  Bus Creator1/1 -> Switch1/1
  Charger_U2/1 -> Bus Creator2/1
  Charger_I2/1 -> Bus Creator2/2
  Bus Creator2/1 -> Switch1/3
  Switch1/1 -> Switch/1
  Switch/1 -> Bus Selector/1
  Bus Selector/1 -> ChargerOutputVoltage/1  "<signal1>"
  Bus Selector/2 -> ChargerOutputCurrent/1  "<signal2>"

== system HQEV_MiL_20160830_integrate_2010a/MiL/Test_Integration/Charger/Charger/Charger/Charger/Work/Subsystem/Constant ==
  Constant1 : Constant  Value=30
  Constant2 : Constant
  Constant5 : Constant  Value=0
  ChargerStatus : Outport
  RechargeRequest : Outport  Port=2
  ChargerTemperature : Outport  Port=3
  wires:
  Constant2/1 -> ChargerStatus/1
  Constant5/1 -> RechargeRequest/1
  Constant1/1 -> ChargerTemperature/1

== system HQEV_MiL_20160830_integrate_2010a/MiL/Test_Integration/Driver/Driver/Driver_AutoPedal/CTRL BrakePed/velocoty/Run_Forward/Difference ==
  In1 : Inport
  Sum2 : Sum  Inputs=+-|
  Unit Delay : UnitDelay  SampleTime=-1
  Out1 : Outport
  wires:
  Sum2/1 -> Out1/1  "Gradient"
  In1/1 -> Unit Delay/1, Sum2/1
  Unit Delay/1 -> Sum2/2

== system HQEV_MiL_20160830_integrate_2010a/MiL/Test_Integration/MCU_FF/MCU/MCU/Torque_Control/Subsystem/Max_Torque/Max_Gen_Torque_Subsystem ==
  EM_Volt : Inport
  EM_spd : Inport  Port=2
  Bus Creator : BusCreator  Inputs=3
  Constant : Constant  Value=-1
  Constant1 : Constant  Value=-1
  Constant2 : Constant  Value=-1
  Interpolation_2nd : Subsystem
  Max_Gen_Torque_at_300V : Lookup  InputValues=|  Table=|  LookUpMeth=Interpolation-Use End Values
      InputValues=|
      | [0
      | 500
      | 1000
      | 1500
      | 2000
      | 2500
      | 2700
      | 3000
      | 3500
      | 4000
      | 4500
      | 5000
      | 5500
      | 6000
      | 6500
      | 7000
      | 7500
      | 8000
      | 8500
      | 9000
      | 9500
      | 10000
      | 10500
      | 11000
      | 11500
      | 12000
      | ]
      Table=|
      | [340
      | 340
      | 340
      | 340
      | 340
      | 340
      | 340
      | 316
      | 272
      | 236
      | 206
      | 180
      | 160
      | 144
      | 130
      | 120
      | 110
      | 102
      | 94
      | 88
      | 84
      | 78
      | 74
      | 70
      | 66
      | 64
      | ]
  Max_Gen_Torque_at_340V : Lookup  InputValues=|  Table=|  LookUpMeth=Interpolation-Use End Values
      InputValues=|
      | [0
      | 500
      | 1000
      | 1500
      | 2000
      | 2500
      | 3000
      | 3100
      | 3500
      | 4000
      | 4500
      | 5000
      | 5500
      | 6000
      | 6500
      | 7000
      | 7500
      | 8000
      | 8500
      | 9000
      | 9500
      | 10000
      | 10500
      | 11000
      | 11500
      | 12000
      | ]
      Table=|
      | [340
      | 340
      | 340
      | 340
      | 340
      | 340
      | 340
      | 340
      | 310
      | 272
      | 240
      | 212
      | 190
      | 170
      | 154
      | 140
      | 128
      | 118
      | 110
      | 104
      | 96
      | 90
      | 86
      | 82
      | 78
      | 74
      | ]
  Max_Mot_Torque_at_280V : Lookup  InputValues=|  Table=|  LookUpMeth=Interpolation-Use End Values
      InputValues=|
      | [0
      | 500
      | 1000
      | 1500
      | 2000
      | 2500
      | 3000
      | 3500
      | 4000
      | 4500
      | 5000
      | 5500
      | 6000
      | 6500
      | 7000
      | 7500
      | 8000
      | 8500
      | 9000
      | 9500
      | 10000
      | 10500
      | 11000
      | 11500
      | 12000
      | ]
      Table=|
      | [340
      | 340
      | 340
      | 340
      | 340
      | 340
      | 296
      | 252
      | 218
      | 188
      | 166
      | 146
      | 132
      | 120
      | 110
      | 102
      | 94
      | 88
      | 82
      | 76
      | 72
      | 68
      | 64
      | 62
      | 58
      | ]
  Product : Product  RndMeth=Zero
  Product1 : Product  RndMeth=Zero
  Product2 : Product  RndMeth=Zero
  abs_val : Subsystem
  Out1 : Outport
  wires:
  Interpolation_2nd/1(Out1) -> Out1/1
  EM_spd/1 -> abs_val/1(In1)
  Bus Creator/1 -> Interpolation_2nd/2(In2)
  EM_Volt/1 -> Interpolation_2nd/1(In1)
  abs_val/1(Out1) -> Max_Gen_Torque_at_340V/1, Max_Gen_Torque_at_300V/1, Max_Mot_Torque_at_280V/1
  Max_Mot_Torque_at_280V/1 -> Product/1
  Max_Gen_Torque_at_300V/1 -> Product1/1
  Max_Gen_Torque_at_340V/1 -> Product2/1
  Constant/1 -> Product/2
  Constant1/1 -> Product1/2
  Constant2/1 -> Product2/2
  Product/1 -> Bus Creator/1  "at280V"
  Product1/1 -> Bus Creator/2  "at300V"
  Product2/1 -> Bus Creator/3  "at340V"

== system HQEV_MiL_20160830_integrate_2010a/MiL/Test_Integration/MCU_FF/MCU/MCU/Torque_Control/Subsystem/Max_Torque/Max_Mot_Torque_Subsystem ==
  EM_Volt : Inport
  EM_spd : Inport  Port=2
  Bus Creator : BusCreator  Inputs=3
  Interpolation_2nd : Subsystem
  Max_Gen_Torque_at_300V : Lookup  InputValues=|  Table=|  LookUpMeth=Interpolation-Use End Values
      InputValues=|
      | [0
      | 500
      | 1000
      | 1500
      | 2000
      | 2500
      | 2700
      | 3000
      | 3500
      | 4000
      | 4500
      | 5000
      | 5500
      | 6000
      | 6500
      | 7000
      | 7500
      | 8000
      | 8500
      | 9000
      | 9500
      | 10000
      | 10500
      | 11000
      | 11500
      | 12000
      | ]
      Table=|
      | [340
      | 340
      | 340
      | 340
      | 340
      | 340
      | 340
      | 316
      | 272
      | 236
      | 206
      | 180
      | 160
      | 144
      | 130
      | 120
      | 110
      | 102
      | 94
      | 88
      | 84
      | 78
      | 74
      | 70
      | 66
      | 64
      | ]
  Max_Gen_Torque_at_340V : Lookup  InputValues=|  Table=|  LookUpMeth=Interpolation-Use End Values
      InputValues=|
      | [0
      | 500
      | 1000
      | 1500
      | 2000
      | 2500
      | 3000
      | 3100
      | 3500
      | 4000
      | 4500
      | 5000
      | 5500
      | 6000
      | 6500
      | 7000
      | 7500
      | 8000
      | 8500
      | 9000
      | 9500
      | 10000
      | 10500
      | 11000
      | 11500
      | 12000
      | ]
      Table=|
      | [340
      | 340
      | 340
      | 340
      | 340
      | 340
      | 340
      | 340
      | 310
      | 272
      | 240
      | 212
      | 190
      | 170
      | 154
      | 140
      | 128
      | 118
      | 110
      | 104
      | 96
      | 90
      | 86
      | 82
      | 78
      | 74
      | ]
  Max_Mot_Torque_at_280V : Lookup  InputValues=|  Table=|  LookUpMeth=Interpolation-Use End Values
      InputValues=|
      | [0
      | 500
      | 1000
      | 1500
      | 2000
      | 2500
      | 3000
      | 3500
      | 4000
      | 4500
      | 5000
      | 5500
      | 6000
      | 6500
      | 7000
      | 7500
      | 8000
      | 8500
      | 9000
      | 9500
      | 10000
      | 10500
      | 11000
      | 11500
      | 12000
      | ]
      Table=|
      | [340
      | 340
      | 340
      | 340
      | 340
      | 340
      | 296
      | 252
      | 218
      | 188
      | 166
      | 146
      | 132
      | 120
      | 110
      | 102
      | 94
      | 88
      | 82
      | 76
      | 72
      | 68
      | 64
      | 62
      | 58
      | ]
  abs_val : Subsystem
  Out1 : Outport
  wires:
  abs_val/1(Out1) -> Max_Mot_Torque_at_280V/1, Max_Gen_Torque_at_300V/1, Max_Gen_Torque_at_340V/1
  Max_Mot_Torque_at_280V/1 -> Bus Creator/1  "at280V"
  Max_Gen_Torque_at_300V/1 -> Bus Creator/2  "at300V"
  Max_Gen_Torque_at_340V/1 -> Bus Creator/3  "at340V"
  EM_Volt/1 -> Interpolation_2nd/1(In1)
  Bus Creator/1 -> Interpolation_2nd/2(In2)
  EM_spd/1 -> abs_val/1(In1)
  Interpolation_2nd/1(Out1) -> Out1/1

== system HQEV_MiL_20160830_integrate_2010a/MiL/Test_Integration/MCU_RR/MCU/MCU/Subsystem14/Rapid_Discharge/Subsystem/Subsystem ==
  EM_spd : Inport
  Constant : Constant  Value=170
  Constant1 : Constant  Value=0
  Constant2 : Constant
  Relational Operator : RelationalOperator  Operator=<  LogicOutDataTypeMode=boolean  OutDataTypeStr=boolean
  Switch : Switch  Criteria=u2 ~= 0
  PWM : Outport
  wires:
  EM_spd/1 -> Relational Operator/1
  Constant/1 -> Relational Operator/2
  Relational Operator/1 -> Switch/2
  Constant1/1 -> Switch/1
  Constant2/1 -> Switch/3
  Switch/1 -> PWM/1

== system HQEV_MiL_20160830_integrate_2010a/MiL/Test_Integration/MCU_RR/MCU/MCU/Subsystem14/Standby/Subsystem/Subsystem ==
  EM_spd : Inport
  Constant : Constant  Value=170
  Constant1 : Constant  Value=0
  Constant2 : Constant
  Relational Operator : RelationalOperator  Operator=<  LogicOutDataTypeMode=boolean  OutDataTypeStr=boolean
  Switch : Switch  Criteria=u2 ~= 0
  PWM : Outport
  wires:
  EM_spd/1 -> Relational Operator/1
  Constant/1 -> Relational Operator/2
  Relational Operator/1 -> Switch/2
  Constant1/1 -> Switch/1
  Constant2/1 -> Switch/3
  Switch/1 -> PWM/1

== system HQEV_MiL_20160830_integrate_2010a/MiL/Test_Integration/MCU_RR/MCU/MCU/Subsystem14/Stop/Subsystem/Subsystem ==
  EM_spd : Inport
  Constant : Constant  Value=170
  Constant1 : Constant  Value=0
  Constant2 : Constant
  Relational Operator : RelationalOperator  Operator=<  LogicOutDataTypeMode=boolean  OutDataTypeStr=boolean
  Switch : Switch  Criteria=u2 ~= 0
  PWM : Outport
  wires:
  EM_spd/1 -> Relational Operator/1
  Constant/1 -> Relational Operator/2
  Relational Operator/1 -> Switch/2
  Constant1/1 -> Switch/1
  Constant2/1 -> Switch/3
  Switch/1 -> PWM/1

== system HQEV_MiL_20160830_integrate_2010a/MiL/Test_Integration/MCU_RR/MCU/MCU/Subsystem14/Torque_Control/Subsystem/Max_Torque ==
  EM_Volt : Inport
  EM_spd : Inport  Port=2
  Max_Gen_Torque_Subsystem : Subsystem
  Max_Mot_Torque_Subsystem : Subsystem
  Unit Delay : UnitDelay  SampleTime=-1
  Unit Delay1 : UnitDelay  SampleTime=-1
  Max_Mot_Torque : Outport
  Max_Gen_Torque : Outport  Port=2
  wires:
  EM_spd/1 -> Max_Mot_Torque_Subsystem/2(EM_spd), Max_Gen_Torque_Subsystem/2(EM_spd)
  Max_Mot_Torque_Subsystem/1(Out1) -> Unit Delay/1
  EM_Volt/1 -> Max_Mot_Torque_Subsystem/1(EM_Volt), Max_Gen_Torque_Subsystem/1(EM_Volt)
  Max_Gen_Torque_Subsystem/1(Out1) -> Unit Delay1/1
  Unit Delay/1 -> Max_Mot_Torque/1
  Unit Delay1/1 -> Max_Gen_Torque/1

== system HQEV_MiL_20160830_integrate_2010a/MiL/Test_Integration/Motor_FF/Motor/Motor/eMotor/Electric Power/Motor Electric Power/abs ==
  In1 : Inport
  Constant : Constant  Value=-1
  Divide3 : Product  Inputs=**
  Switch1 : Switch  Criteria=u2 > Threshold
  Out1 : Outport
  wires:
  Constant/1 -> Divide3/2
  Divide3/1 -> Switch1/3
  In1/1 -> Divide3/1, Switch1/2, Switch1/1
  Switch1/1 -> Out1/1

== system HQEV_MiL_20160830_integrate_2010a/MiL/Test_Integration/Motor_FF/Motor/Motor/eMotor/Electric Power/Motor Electric Power/abs1 ==
  In1 : Inport
  Constant : Constant  Value=-1
  Divide3 : Product  Inputs=**
  Switch1 : Switch  Criteria=u2 > Threshold
  Out1 : Outport
  wires:
  Switch1/1 -> Out1/1
  In1/1 -> Switch1/1, Switch1/2, Divide3/1
  Divide3/1 -> Switch1/3
  Constant/1 -> Divide3/2

== system HQEV_MiL_20160830_integrate_2010a/MiL/Test_Integration/Motor_FF/Motor/Motor/eMotor/Electric Power/Motor Electric Power/abs2 ==
  In1 : Inport
  Constant : Constant  Value=-1
  Divide3 : Product  Inputs=**
  Switch1 : Switch  Criteria=u2 > Threshold
  Out1 : Outport
  wires:
  Switch1/1 -> Out1/1
  In1/1 -> Switch1/1, Switch1/2, Divide3/1
  Divide3/1 -> Switch1/3
  Constant/1 -> Divide3/2

== system HQEV_MiL_20160830_integrate_2010a/MiL/Test_Integration/Motor_RR/Motor/Motor1/eMotor/Electric Power/Motor Electric Power/abs ==
  In1 : Inport
  Constant : Constant  Value=-1
  Divide3 : Product  Inputs=**
  Switch1 : Switch  Criteria=u2 > Threshold
  Out1 : Outport
  wires:
  Constant/1 -> Divide3/2
  Divide3/1 -> Switch1/3
  In1/1 -> Divide3/1, Switch1/2, Switch1/1
  Switch1/1 -> Out1/1

== system HQEV_MiL_20160830_integrate_2010a/MiL/Test_Integration/Motor_RR/Motor/Motor1/eMotor/Electric Power/Motor Electric Power/abs1 ==
  In1 : Inport
  Constant : Constant  Value=-1
  Divide3 : Product  Inputs=**
  Switch1 : Switch  Criteria=u2 > Threshold
  Out1 : Outport
  wires:
  Switch1/1 -> Out1/1
  In1/1 -> Switch1/1, Switch1/2, Divide3/1
  Divide3/1 -> Switch1/3
  Constant/1 -> Divide3/2

== system HQEV_MiL_20160830_integrate_2010a/MiL/Test_Integration/Motor_RR/Motor/Motor1/eMotor/Electric Power/Motor Electric Power/abs2 ==
  In1 : Inport
  Constant : Constant  Value=-1
  Divide3 : Product  Inputs=**
  Switch1 : Switch  Criteria=u2 > Threshold
  Out1 : Outport
  wires:
  Switch1/1 -> Out1/1
  In1/1 -> Switch1/1, Switch1/2, Divide3/1
  Divide3/1 -> Switch1/3
  Constant/1 -> Divide3/2

== system HQEV_MiL_20160830_integrate_2010a/MiL/Test_Integration/MCU_FF/MCU/MCU/Torque_Control/Subsystem/Max_Torque/Max_Gen_Torque_Subsystem/Interpolation_2nd ==
  In1 : Inport
  In2 : Inport  Port=2
  0V_280V : Subsystem
  280V_300V : Subsystem
  300V_340V : Subsystem
  340V_inf : Subsystem
  MM : Subsystem
  Multiport Switch : MultiPortSwitch  Inputs=4  zeroidx=off
  Out1 : Outport
  wires:
  In2/1 -> 300V_340V/2(In2), 340V_inf/1(In1), 280V_300V/2(In2), 0V_280V/1(In1)
  Multiport Switch/1 -> Out1/1
  MM/1(Out1) -> Multiport Switch/1
  In1/1 -> 300V_340V/1(In1), 280V_300V/1(In1), MM/1(In1)
  340V_inf/1(Out1) -> Multiport Switch/5
  300V_340V/1(Out1) -> Multiport Switch/4
  280V_300V/1(Out1) -> Multiport Switch/3
  0V_280V/1(Out1) -> Multiport Switch/2

== system HQEV_MiL_20160830_integrate_2010a/MiL/Test_Integration/MCU_FF/MCU/MCU/Torque_Control/Subsystem/Max_Torque/Max_Gen_Torque_Subsystem/abs_val ==
  In1 : Inport
  Constant : Constant  Value=0
  Constant1 : Constant  Value=-1
  Product : Product  RndMeth=Zero
  Relational Operator : RelationalOperator  LogicOutDataTypeMode=boolean  OutDataTypeStr=boolean
  Switch : Switch  Criteria=u2 ~= 0
  Out1 : Outport
  wires:
  Switch/1 -> Out1/1
  In1/1 -> Product/1, Relational Operator/1, Switch/1
  Constant1/1 -> Product/2
  Product/1 -> Switch/3
  Relational Operator/1 -> Switch/2
  Constant/1 -> Relational Operator/2

== system HQEV_MiL_20160830_integrate_2010a/MiL/Test_Integration/MCU_FF/MCU/MCU/Torque_Control/Subsystem/Max_Torque/Max_Mot_Torque_Subsystem/Interpolation_2nd ==
  In1 : Inport
  In2 : Inport  Port=2
  0V_280V : Subsystem
  280V_300V : Subsystem
  300V_340V : Subsystem
  340V_inf : Subsystem
  MM : Subsystem
  Multiport Switch : MultiPortSwitch  Inputs=4  zeroidx=off
  Out1 : Outport
  wires:
  0V_280V/1(Out1) -> Multiport Switch/2
  280V_300V/1(Out1) -> Multiport Switch/3
  300V_340V/1(Out1) -> Multiport Switch/4
  340V_inf/1(Out1) -> Multiport Switch/5
  In1/1 -> MM/1(In1), 280V_300V/1(In1), 300V_340V/1(In1)
  MM/1(Out1) -> Multiport Switch/1
  Multiport Switch/1 -> Out1/1
  In2/1 -> 0V_280V/1(In1), 280V_300V/2(In2), 340V_inf/1(In1), 300V_340V/2(In2)

== system HQEV_MiL_20160830_integrate_2010a/MiL/Test_Integration/MCU_FF/MCU/MCU/Torque_Control/Subsystem/Max_Torque/Max_Mot_Torque_Subsystem/abs_val ==
  In1 : Inport
  Constant : Constant  Value=0
  Constant1 : Constant  Value=-1
  Product : Product  RndMeth=Zero
  Relational Operator : RelationalOperator  LogicOutDataTypeMode=boolean  OutDataTypeStr=boolean
  Switch : Switch  Criteria=u2 ~= 0
  Out1 : Outport
  wires:
  Constant/1 -> Relational Operator/2
  Relational Operator/1 -> Switch/2
  Product/1 -> Switch/3
  Constant1/1 -> Product/2
  In1/1 -> Switch/1, Relational Operator/1, Product/1
  Switch/1 -> Out1/1
